simulink model "adaptive"  (R2018b)
settings: Solver=VariableStepAuto  StartTime=0.0  StopTime=40  RelTol=1e-3
values from neighbouring files (symbols this model uses):
  ADAMS_cwd = 'C:\adams_work\three_dof'    [Controls_Plant_1.m]
  ADAMS_exec = ''    [Controls_Plant_1.m]
  ADAMS_host = 'LAPTOP-5088IVHI'    [Controls_Plant_1.m]
  ADAMS_init = ''    [Controls_Plant_1.m]
  ADAMS_inputs = 'torque1!torque2!torque3'    [Controls_Plant_1.m]
  ADAMS_outputs = 'q1m!q2m!q3m!v1!v2!v3!a1!a2!a3'    [Controls_Plant_1.m]
  ADAMS_prefix = 'Controls_Plant_1'    [Controls_Plant_1.m]
  ADAMS_static = 'no'    [Controls_Plant_1.m]
  ADAMS_sysdir = 'C:\ruanjian\Adams\'    [Controls_Plant_1.m]
settings Model: Creator=73514  LastModifiedBy=73514

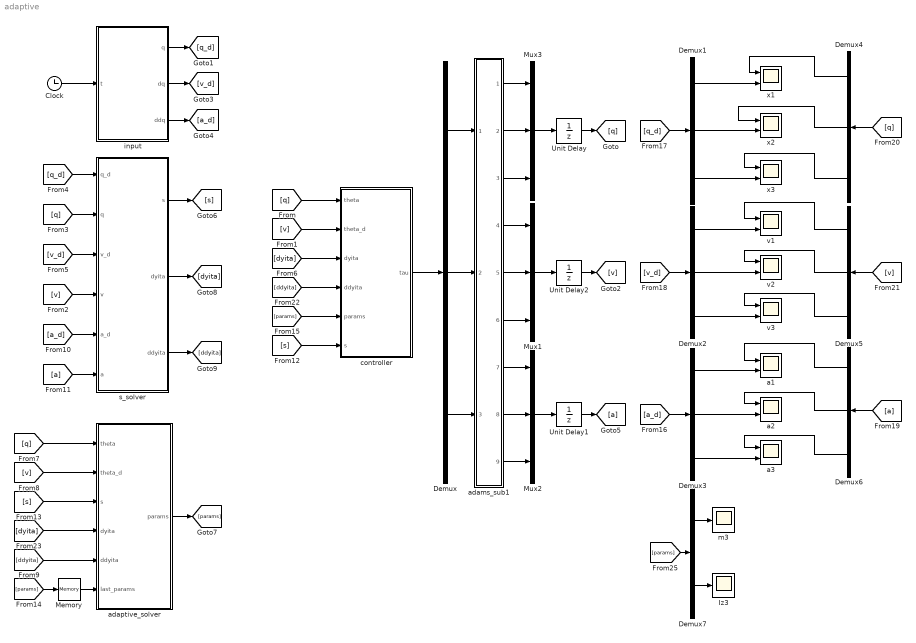
== system adaptive ==
  Clock : Clock
  Demux{,1..6} (7 alike) : Demux  Outputs=3
  Demux7 : Demux  Outputs=2
  Iz3 : Scope
  Memory : Memory  InitialCondition=[8,2]
  Mux1 : Mux  Inputs=3
  Mux2 : Mux  Inputs=3
  Mux3 : Mux  Inputs=3
  Unit Delay : UnitDelay  SampleTime=-1
  Unit Delay1 : UnitDelay  SampleTime=-1
  Unit Delay2 : UnitDelay  SampleTime=-1
  a1 : Scope  NumInputPorts=2
  a2 : Scope  NumInputPorts=2
  a3 : Scope  NumInputPorts=2
  adams_sub1 : Subsystem
  adaptive_solver : MATLAB Function  TreatAsAtomicUnit=on
  controller : MATLAB Function  TreatAsAtomicUnit=on
  input : MATLAB Function  TreatAsAtomicUnit=on
  m3 : Scope
  "s_solver " : MATLAB Function  TreatAsAtomicUnit=on
  v1 : Scope  NumInputPorts=2
  v2 : Scope  NumInputPorts=2
  v3 : Scope  NumInputPorts=2
  x1 : Scope  NumInputPorts=2
  x2 : Scope  NumInputPorts=2
  x3 : Scope  NumInputPorts=2
  wires:
  Unit Delay/1 -> [q]
  [q] -> controller/1(theta)
  Mux1/1 -> Unit Delay2/1
  Unit Delay2/1 -> [v]
  controller/1(tau) -> Demux/1
  Mux3/1 -> Unit Delay/1
  Demux/1 -> adams_sub1/1(torque1)
  [v] -> controller/2(theta_d)
  input/1(q) -> [q_d]
  input/3(ddq) -> [a_d]
  input/2(dq) -> [v_d]
  [dyita] -> controller/3(dyita)
  [q] -> adaptive_solver/1(theta)
  [v] -> adaptive_solver/2(theta_d)
  Unit Delay1/1 -> [a]
  Mux2/1 -> Unit Delay1/1
  [dyita] -> adaptive_solver/4(dyita)
  Clock/1 -> input/1(t)
  [q_d] -> "s_solver "/1(q_d)
  [q] -> "s_solver "/2(q)
  [v_d] -> "s_solver "/3(v_d)
  [v] -> "s_solver "/4(v)
  [a_d] -> "s_solver "/5(a_d)
  [a] -> "s_solver "/6(a)
  "s_solver "/1(s) -> [s]
  [s] -> controller/6(s)
  [s] -> adaptive_solver/3(s)
  adaptive_solver/1(params) -> [params]
  [params] -> controller/5(params)
  [params] -> Memory/1
  Memory/1 -> adaptive_solver/6(last_params)
  Demux/2 -> adams_sub1/2(torque2)
  Demux/3 -> adams_sub1/3(torque3)
  [v_d] -> Demux2/1
  [a_d] -> Demux3/1
  [q_d] -> Demux1/1
  adams_sub1/1(q1m) -> Mux3/1
  adams_sub1/2(q2m) -> Mux3/2
  adams_sub1/3(q3m) -> Mux3/3
  adams_sub1/4("v1 ") -> Mux1/1
  adams_sub1/5("v2 ") -> Mux1/2
  adams_sub1/6("v3 ") -> Mux1/3
  adams_sub1/7("a1 ") -> Mux2/1
  adams_sub1/8("a2 ") -> Mux2/2
  adams_sub1/9("a3 ") -> Mux2/3
  [v] -> Demux5/1
  [q] -> Demux4/1
  [a] -> Demux6/1
  Demux1/1 -> x1/2
  Demux1/2 -> x2/2
  Demux1/3 -> x3/2
  Demux2/1 -> v1/2
  Demux2/2 -> v2/2
  Demux2/3 -> v3/2
  Demux3/1 -> a1/2
  Demux3/2 -> a2/2
  Demux3/3 -> a3/2
  Demux4/1 -> x1/1
  Demux4/2 -> x2/1
  Demux4/3 -> x3/1
  Demux5/1 -> v1/1
  Demux5/2 -> v2/1
  Demux5/3 -> v3/1
  Demux6/1 -> a1/1
  Demux6/2 -> a2/1
  Demux6/3 -> a3/1
  "s_solver "/2(dyita) -> [dyita]
  "s_solver "/3(ddyita) -> [ddyita]
  [ddyita] -> controller/4(ddyita)
  [ddyita] -> adaptive_solver/5(ddyita)
  [params] -> Demux7/1
  Demux7/1 -> m3/1
  Demux7/2 -> Iz3/1

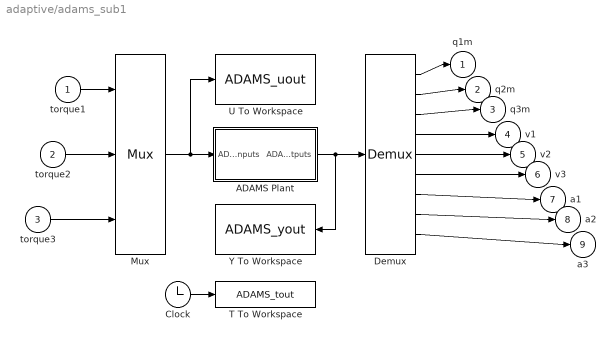
== system adaptive/adams_sub1 ==
  torque1 : Inport
  torque2 : Inport  Port=2
  torque3 : Inport  Port=3
  ADAMS Plant : Subsystem  LoadFcn=|  InitFcn=clear mex  mask(Adams Plant){exevie=ADAMS_sysdir, nam_in=ADAMS_inputs, namout=ADAMS_outputs, nampre=ADAMS_prefix, outfil=ADAMS_prefix, exesol=ADAMS_exec, stat=ADAMS_static, inicmd=[ADAMS_init], exetyp=C++, comtyp=PIPE(DDE), workdir=ADAMS_cwd, ada_host=ADAMS_host, modani=batch, modsim=discrete, dft=no, simulink_lead_cosim=yes, pin_interp_order=0, pout_extrap_order=0, pin_extrap_order=0, pout_interp_order=0, dt_out=0.005, o_rate=1, more=off}
      | %check based on dialog box setting for when setting by popup menu                                             
      | if exist('ADAMS_solver_type')                                                                                 
      |   if strcmp(ADAMS_solver_type,'C++')                                                                          
      |     set_param(gcb,'exetyp','C++');                                                                            
      |   else                                                                                                        
      |     set_param(gcb,'exetyp','Fortran');                                                                        
      |   end                                                                                                         
      | else                                                                                                          
      |   set_param(gcb,'exetyp','C++');                                                                              
      | end                                                                                                           
      | %set the mode if using acar_solver                                                                            
      | %REQUIRED HERE BECAUSE BELOW CAUSES MDLTERMINATE TO BE CALLED 2 TIMES IN MIDDLE OF SIMULATION WHEN SET IN MASK
      |                                                                                                               
      | %enable the direct feedthrough, sim mode, anim mode parameters by default                                     
      |                                                                                                               
      | if exist('set_some_params_states')                                                                            
      |                                                                                                               
      |   set_some_params_states({'dft','modsim','modani'},{'on','on','on'},'MaskEnables',gcb)                        
      |   %turn on direct feedthrough option                                                                          
      |   set_some_params_states({'dft'},{'on'},'MaskVisibilities',gcb)                                               
      |                                                                                                               
      |  end                                                                                                          
      |                                                                                                               
      |                                                                                                               
      | if exist('ADAMS_exec')                                                                                        
      |   if and(strcmp(get_param(gcb,'exesol'),'ADAMS_exec'),strcmp(ADAMS_exec,'acar_solver'))                       
      |     %set the sim mode to discrete -- only supported mode                                                      
      |     set_param(gcb,'modsim','discrete')                                                                        
      |      %turn off direct feedthrough option                                                                      
      |      set_some_params_states({'dft'},{'off'},'MaskVisibilities',gcb)                                           
      |     %set the animation mode to batch -- only supported mode                                                   
      |     set_param(gcb,'modani','batch')                                                                           
      |     %disable the direct feedthrough, sim mode, anim mode parameters                                           
      |     set_some_params_states({'modsim','modani'},{'off','off'},'MaskEnables',gcb)                               
      |   end
      |   if and(strcmp(get_param(gcb,'exesol'),'ADAMS_exec'),strcmp(ADAMS_exec,'apre_solver'))                       
      |     %set the sim mode to discrete -- only supported mode                                                      
      |     set_param(gcb,'modsim','discrete')                                                                        
      |      %turn off direct feedthrough option                                                                      
      |      set_some_params_states({'dft'},{'off'},'MaskVisibilities',gcb)                                           
      |     %set the animation mode to batch -- only supported mode                                                   
      |     set_param(gcb,'modani','batch')                                                                           
      |     %disable the direct feedthrough, sim mode, anim mode parameters                                           
      |     set_some_params_states({'modsim','modani'},{'off','off'},'MaskEnables',gcb)                               
      |   end                                                                                                  
      | end
      mask prompts: exevie "Adams install directory"; nam_in "Adams View input names"; namout "Adams View output names"; nampre "Adams model file prefix"; outfil "Output files prefix (opt.: if blank - no output)"; exesol "User executable (opt.: if blank - use standard)"; stat "Initial static simulation flag"; inicmd "Initialization commands"; exetyp "Adams Solver type"; comtyp "Interprocess option"; workdir "Adams working directory"; ada_host "Adams host"; modani "Animation mode"; modsim "Simulation mode"; dft "Direct feedthrough"; simulink_lead_cosim "Discrete Computational Order - Simulink Leads Adams"; pin_interp_order "Plant input interpolation order"; pout_extrap_order "Plant output extrapolation order"; pin_extrap_order "Plant input extrapolation order"; pout_interp_order "Plant output interpolation order"; dt_out "Communication interval"; o_rate "Number of communications per output step"; more "More parameters"
      mask help: Simulate any Adams plant model either in Adams Solver form (.adm file) or in Adams View form (.cmd file)
      settings: OpenFcn=|
      | open_system(gcb,'mask')
      | if not(exist('set_some_params_states'))
      | 
      | warning('The script "set_some_params_states.m" cannot be found in the MATLAB PATH.  Cannot update the ADAMS Plant S-Function parameters.')
      | 
      | warning('Recommended action(optional):  run the Adams Controls .m file first to help choose the correct settings in the Adams S-Function block.')
      | 
      | end
      mask Help:
      | <html>
      | This S-Function represents the non-linear Adams Plant with the inputs sent to the Adams model <br>
      |  and the outputs generated by the Adams model.  See the Adams Controls documentation for more <br>
      | information.  This plant uses the following variables:<br>
      | <br>
      | <b>ADAMS_sysdir  :</b> Adams installation directory<br>
      | <b>ADAMS_inputs  :</b> Input variables View names vector<br>
      | <b>ADAMS_outputs :</b> Outputs variables View names vector<br>
      | <b>ADAMS_prefix  : </b>ADAMS model files prefix (.adm, .cmd); also doubles as output files prefix<br>
      | <b>ADAMS_exec :</b> Adams Solver user library or keyword (e.g., acar_solver)<br>
      | <b>ADAMS_static :</b> yes|no - initial static before Co-simulation(discrete)/Function Evaluation(continuous)<br>
      | <b>ADAMS_init :</b>Initialization commands (i.e., Adams View or Solver commands, depending on setting for Animation mode)<br>
      | <b>ADAMS_cwd : </b> Current working directory (for TCP/IP)<br>
      | <b>ADAMS_host : </b>Name of Adams server host (for TCP/IP)<br>
      | <b>ADAMS_mode :</b> Linear or non-linear (i.e., co-sim, function eval)<br>
      | <b>ADAMS_solver_type :</b>Fortran or C++ (used to set popup menu when first loaded) <br>
      | 
      | 
      | <br>
      | The following settings can be chosen:<br>
      | <br>
      | <b>Adams Solver type:</b>  Fortran or C++ (will also set ADAMS_solver_type)<br>
      | <b>Interprocess option:</b> Pipe(DDE), TCP/IP or DIRECT; TCP/IP can allow different machines run Adams and MATLAB<br>
      | <b>Animation mode:</b> batch (Solver, uses .adm) or interactive (View, uses .cmd)<br>
      | <b>Simulation mode:</b> discrete (Co-simulation) or continuous (Function Evaluation)<br>
      | <b>Discrete Computational Order - Simulink Lead Adams:</b> for discrete mode, chooses if Simulink leads the integration (yes) or lags (no);<br> if set to "no", can remove algebraic loop<br>
      | <b>Plant input interpolation order:</b> 0 = zero-order hold; 1 = linear (discrete mode only, where Simulink leads)<br>
      | <b>Plant output extrapolation order:</b> 0 = zero-order hold;1 = linear(discrete mode only, where Simulink leads)<br>
      | <b>Plant input extrapolation order:</b> 0 = zero-order hold; 1 = linear (discrete mode only, where Adams leads)<br>
      | <b>Plant output interpolation order:</b> 0 = zero-order hold;1 = linear(discrete mode only, where Adams leads)<br>
      | <b>Direct feedthrough:</b> yes|no - yes = Input directly effect output(continuous mode-only)<br>
      | <b>Communication interval:</b> Time step at which Co-simulation exchange information (e.g.,0.005); also controls <br>output for continuous mode (Function Evaluation)<br>
      | <b>Number of communications per output step: </b>Sets Adams output rate (.res, .req, .gra) integer value (default: 1)<br>
      | </html>
      mask Callback exesol:
      | if exist('set_some_params_states')
      | %enable the direct feedthrough, sim mode, anim mode parameters
      | set_some_params_states({'dft','modsim','modani'},{'on','on','on'},'MaskEnables',gcb)
      | %turn on direct feedthrough option
      | set_some_params_states({'dft'},{'on'},'MaskVisibilities',gcb)
      | end
      | 
      | if exist('ADAMS_exec')
      |   if and(strcmp(get_param(gcb,'exesol'),'ADAMS_exec'),strcmp(ADAMS_exec,'acar_solver'))
      |     %set the sim mode to discrete -- only supported mode
      |     %REMOVED:  BELOW CAUSES MDLTERMINATE TO BE CALLED 2 TIMES IN MIDDLE OF SIMULATION
      |     %Now in LoadFcn callback
      |     %set_param(gcb,'modsim','discrete')
      |      %turn off direct feedthrough option
      |     set_some_params_states({'dft'},{'off'},'MaskVisibilities',gcb)
      |     %set the animation mode to batch -- only supported mode
      |     %REMOVED:  BELOW CAUSES MDLTERMINATE TO BE CALLED 2 TIMES IN MIDDLE OF SIMULATION
      |     %Now in LoadFcn callback
      |     %set_param(gcb,'modani','batch')
      |     %disable the direct feedthrough, sim mode, anim mode parameters
      |     set_some_params_states({'modsim','modani'},{'off','off'},'MaskEnables',gcb)
      |   end
      | end
      mask TypeOptions exetyp: Fortran | C++
      mask Callback exetyp:
      | if strcmp(get_param(gcb,'exetyp'),'C++')
      |     ADAMS_solver_type='C++';
      | else
      |     ADAMS_solver_type='Fortran';
      | end
      mask TypeOptions comtyp: PIPE(DDE) | TCP/IP | DIRECT
      mask Callback comtyp:
      | if exist('set_some_params_states')
      | if strcmp(get_param(gcb,'comtyp'),'PIPE(DDE)') || strcmp(get_param(gcb,'comtyp'),'DIRECT')
      |     %turn off cwd, host options
      |     set_some_params_states({'ada_host','workdir'},{'off','off'},'MaskVisibilities',gcb)
      | else%if strcmp(get_param(gcb,'modsim'),'TCP/IP')
      |     %turn on cwd, host options
      |     set_some_params_states({'ada_host','workdir'},{'on','on'},'MaskVisibilities',gcb)
      | end
      | end
      mask TypeOptions modani: batch | interactive
      mask TypeOptions modsim: discrete | continuous
      mask Callback modsim:
      | if exist('set_some_params_states')
      | if strcmp(get_param(gcb,'modsim'),'discrete')
      |      %turn off direct feedthrough option
      |     set_some_params_states({'dft'},{'off'},'MaskVisibilities',gcb)
      |     %turn on discrete co-sim type if want to see more
      |     if strcmp(get_param(gcb,'more'),'on')
      |         set_some_params_states({'simulink_lead_cosim'},{'on'},'MaskVisibilities',gcb)
      |     end
      |     if strcmp(get_param(gcb,'simulink_lead_cosim'),'yes')
      |         %turn on interpolation/extrapolation options
      |         set_some_params_states({'pin_interp_order','pout_extrap_order',},{'on','on'},'MaskVisibilities',gcb)
      |     else
      |         set_some_params_states({'pin_extrap_order','pout_interp_order'},{'on','on'},'MaskVisibilities',gcb)
      |     end
      | else%if strcmp(get_param(gcb,'modsim'),'continuous')
      |      %turn off direct feedthrough option
      |     set_some_params_states({'dft'},{'on'},'MaskVisibilities',gcb)
      |     %turn off interpolation/extrapolation options
      |     set_some_params_states({'pin_interp_order','pout_extrap_order','pin_extrap_order','pout_interp_order','simulink_lead_cosim'},{'off','off','off','off','off'},'MaskVisibilities',gcb)
      | end
      | end
      mask TypeOptions dft: no | yes
      mask TypeOptions simulink_lead_cosim: yes | no
      mask Callback simulink_lead_cosim:
      | if exist('set_some_params_states')
      | if (strcmp(get_param(gcb,'simulink_lead_cosim'),'yes') && strcmp(get_param(gcb,'modsim'),'discrete'))
      |      %turn off unused interpolate/extrapolate options
      |     set_some_params_states({'pin_extrap_order','pout_interp_order'},{'off','off'},'MaskVisibilities',gcb)
      |     %turn on used interpolate/extrapolate options
      |     set_some_params_states({'pin_interp_order','pout_extrap_order'},{'on','on'},'MaskVisibilities',gcb)
      | elseif (strcmp(get_param(gcb,'simulink_lead_cosim'),'no') && strcmp(get_param(gcb,'modsim'),'discrete'))
      |     %turn on used interpolate/extrapolate options
      |     set_some_params_states({'pin_extrap_order','pout_interp_order'},{'on','on'},'MaskVisibilities',gcb)
      |      %turn off unused interpolate/extrapolate options
      |     set_some_params_states({'pin_interp_order','pout_extrap_order'},{'off','off'},'MaskVisibilities',gcb)
      | end
      | end
      mask TypeOptions pin_interp_order: 0 | 1
      mask TypeOptions pout_extrap_order: 0 | 1
      mask TypeOptions pin_extrap_order: 0 | 1
      mask TypeOptions pout_interp_order: 0 | 1
      mask Callback more:
      | if exist('set_some_params_states')
      | if (strcmp(get_param(gcb,'more'),'on'))
      |      %turn on infrequently used options
      |     set_some_params_states({'exevie','nam_in','namout','exesol','stat','inicmd'},{'on','on','on','on','on','on'},'MaskVisibilities',gcb)
      |     if strcmp(get_param(gcb,'modsim'),'discrete')
      |         set_some_params_states({'simulink_lead_cosim'},{'on'},'MaskVisibilities',gcb)
      |     end
      | elseif (strcmp(get_param(gcb,'more'),'off'))
      |     %turn off infrequently used options
      |     set_some_params_states({'exevie','nam_in','namout','exesol','stat','inicmd'},{'off','off','off','off','off','off'},'MaskVisibilities',gcb)
      |     if strcmp(get_param(gcb,'modsim'),'discrete')
      |         set_some_params_states({'simulink_lead_cosim'},{'off'},'MaskVisibilities',gcb)
      |     end
      | end
      | end
      mask Display: disp( 'MSC Software' )
  Clock : Clock
  Demux : Demux  Outputs=9
  Mux : Mux  Inputs=3
  T To Workspace : ToWorkspace  VariableName=ADAMS_tout
      settings: MaxDataPoints=100000
  U To Workspace : ToWorkspace  VariableName=ADAMS_uout
      settings: MaxDataPoints=100000
  Y To Workspace : ToWorkspace  VariableName=ADAMS_yout
      settings: MaxDataPoints=100000
  q1m : Outport
  q2m : Outport  Port=2
  q3m : Outport  Port=3
  "v1 " : Outport  Port=4
  "v2 " : Outport  Port=5
  "v3 " : Outport  Port=6
  "a1 " : Outport  Port=7
  "a2 " : Outport  Port=8
  "a3 " : Outport  Port=9
  wires:
  Clock/1 -> T To Workspace/1
  Mux/1 -> ADAMS Plant/1(ADAMS inputs), U To Workspace/1
  ADAMS Plant/1(ADAMS outputs) -> Demux/1, Y To Workspace/1
  Demux/1 -> q1m/1
  Demux/2 -> q2m/1
  Demux/3 -> q3m/1
  Demux/4 -> "v1 "/1
  Demux/5 -> "v2 "/1
  Demux/6 -> "v3 "/1
  Demux/7 -> "a1 "/1
  Demux/8 -> "a2 "/1
  Demux/9 -> "a3 "/1
  torque1/1 -> Mux/1
  torque2/1 -> Mux/2
  torque3/1 -> Mux/3

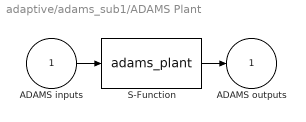
== system adaptive/adams_sub1/ADAMS Plant ==
  ADAMS inputs : Inport
  S-Function : S-Function  StopFcn=clear mex  FunctionName=adams_plant  Parameters=exevie,exesol,stat,outfil,nampre,o_rate,nam_in,namout,dft,modsim,modani,dt_out,inicmd,exetyp,comtyp,ada_host, workdir,pin_interp_order,pout_extrap_order,pin_extrap_order,pout_interp_order,simulink_lead_cosim  SFunctionDeploymentMode=off  EnableBusSupport=off
  ADAMS outputs : Outport  InitialOutput=0
  wires:
  ADAMS inputs/1 -> S-Function/1
  S-Function/1 -> ADAMS outputs/1

== matlab function adaptive/adaptive_solver ==
  data: theta input; params output; theta_d input; s input; dyita input; ddyita input; last_params input
function params = adaptive_solver(theta, theta_d,s,dyita,ddyita,last_params)
dq1=theta_d(1);dq2=theta_d(2);dq3=theta_d(3);
q1=theta(1);q2=theta(2);q3=theta(3);
dyita1=dyita(1);dyita2=dyita(2);dyita3=dyita(3);
ddyita1=ddyita(1);ddyita2=ddyita(2);ddyita3=ddyita(3);
%杆长和质心位置
d1=1; d2=1; d3=1;
xc1=0.5;xc2=0.5;xc3=0.5;
%质量与惯量矩阵
m3=last_params(1);
Iz3=last_params(2);
w=zeros(3,2);
w(1,2)=ddyita1+ddyita2+ddyita3;
w(2,2)=ddyita1+ddyita2+ddyita3;
w(3,2)=ddyita1+ddyita2+ddyita3;
w(1,1)=ddyita3*(d2*xc3*cos(q3) + d1*xc3*cos(q2 + q3)) - dyita2*(d1*dq1*(xc3*sin(q2 + q3) + d2*sin(q2)) + d1*dq2*(xc3*sin(q2 + q3) + d2*sin(q2)) + dq3*xc3*(d1*sin(q2 + q3) + d2*sin(q3))) - dyita1*(dq2*(d1*d2*sin(q2) + d1*xc3*sin(q2 + q3)) + dq3*(d2*xc3*sin(q3) + d1*xc3*sin(q2 + q3))) + ddyita1*(d1^2 + 2*cos(q2)*d1*d2 + 2*xc3*cos(q2 + q3)*d1 + d2^2 + 2*xc3*cos(q3)*d2) + ddyita2*(d2^2 + 2*d2*xc3*cos(q3) + d1*xc3*cos(q2 + q3) + d1*d2*cos(q2)) - dyita3*xc3*(d1*sin(q2 + q3) + d2*sin(q3))*(dq1 + dq2 + dq3);
w(2,1)=dyita1*(dq1*(d1*d2*sin(q2) + d1*xc3*sin(q2 + q3)) - d2*dq3*xc3*sin(q3)) + ddyita1*(d2^2 + 2*d2*xc3*cos(q3) + d1*xc3*cos(q2 + q3) + d1*d2*cos(q2)) + ddyita2*(d2^2 + 2*xc3*cos(q3)*d2) + d2*ddyita3*xc3*cos(q3) - d2*dyita3*xc3*sin(q3)*(dq1 + dq2 + dq3) - d2*dq3*dyita2*xc3*sin(q3);
w(3,1)=ddyita1*(d2*xc3*cos(q3) + d1*xc3*cos(q2 + q3)) + dyita1*(dq1*(d2*xc3*sin(q3) + d1*xc3*sin(q2 + q3)) + d2*dq2*xc3*sin(q3)) + d2*ddyita2*xc3*cos(q3) + d2*dyita2*xc3*sin(q3)*(dq1 + dq2);
%自适应率
gamma=1;
phi=-gamma*w'*s;
m3=m3-phi(1);
Iz3=Iz3-phi(2);
params=[m3,Iz3];
end

== matlab function adaptive/controller ==
  data: theta input; tau output; theta_d input; dyita input; ddyita input; params input; s input
function tau = controller(theta, theta_d, dyita,ddyita, params, s)
tau=zeros(3,1);
dq1=theta_d(1);dq2=theta_d(2);dq3=theta_d(3);
q1=theta(1);q2=theta(2);q3=theta(3);
%杆长和质心位置
d1=1; d2=1; d3=1;
xc1=0.5;xc2=0.5;xc3=0.5;
%质量与惯量矩阵
m1=10;m2=10;m3=params(1);
Iz1=1.05+m1*xc1^2;Iz2=1.05+m2*xc2^2;Iz3=params(2);
%计算
k=100;

h=[ Iz1 + Iz2 + Iz3 + d1^2*m2 + d1^2*m3 + d2^2*m3 + 2*d1*m3*xc3*cos(q2 + q3) + 2*d1*d2*m3*cos(q2) + 2*d1*m2*xc2*cos(q2) + 2*d2*m3*xc3*cos(q3), Iz2 + Iz3 + d2^2*m3 + d1*m3*xc3*cos(q2 + q3) + d1*d2*m3*cos(q2) + d1*m2*xc2*cos(q2) + 2*d2*m3*xc3*cos(q3), Iz3 + d1*m3*xc3*cos(q2 + q3) + d2*m3*xc3*cos(q3);
                                 Iz2 + Iz3 + d2^2*m3 + d1*m3*xc3*cos(q2 + q3) + d1*d2*m3*cos(q2) + d1*m2*xc2*cos(q2) + 2*d2*m3*xc3*cos(q3),                                                                 m3*d2^2 + 2*m3*xc3*cos(q3)*d2 + Iz2 + Iz3,                          Iz3 + d2*m3*xc3*cos(q3);
                                                                                          Iz3 + d1*m3*xc3*cos(q2 + q3) + d2*m3*xc3*cos(q3),                                                                                   Iz3 + d2*m3*xc3*cos(q3),                                              Iz3];

c=[ - dq3*(d1*m3*xc3*sin(q2 + q3) + d2*m3*xc3*sin(q3)) - dq2*(d1*m3*xc3*sin(q2 + q3) + d1*d2*m3*sin(q2) + d1*m2*xc2*sin(q2)), - d1*dq1*(d2*m3*sin(q2) + m2*xc2*sin(q2) + m3*xc3*sin(q2 + q3)) - d1*dq2*(d2*m3*sin(q2) + m2*xc2*sin(q2) + m3*xc3*sin(q2 + q3)) - dq3*m3*xc3*(d1*sin(q2 + q3) + d2*sin(q3)), -m3*xc3*(d1*sin(q2 + q3) + d2*sin(q3))*(dq1 + dq2 + dq3);
                              dq1*(d1*m3*xc3*sin(q2 + q3) + d1*d2*m3*sin(q2) + d1*m2*xc2*sin(q2)) - d2*dq3*m3*xc3*sin(q3),                                                                                                                                                      -d2*dq3*m3*xc3*sin(q3),                     -d2*m3*xc3*sin(q3)*(dq1 + dq2 + dq3);
                                                 dq1*(d1*m3*xc3*sin(q2 + q3) + d2*m3*xc3*sin(q3)) + d2*dq2*m3*xc3*sin(q3),                                                                                                                                               d2*m3*xc3*sin(q3)*(dq1 + dq2),                                                        0];
tau=h*ddyita+c*dyita+k*s;
end

== matlab function adaptive/input ==
  data: t input; q output; dq output; ddq output
function [q,dq,ddq] = input(t)
q=zeros(3,1);
dq=zeros(3,1);
ddq=zeros(3,1);
%等加速度输入信号
%k=0.01;
%a=2*k;
%v=2*k*t;
%x=k*t^2;
%正弦输入信号
k=0.01;w=3;
x=k*(1-cos(w*t));
v=w*k*sin(w*t);
a=w^2*k*cos(w*t);
q=[x;x;x];
dq=[v;v;v];
ddq=[a;a;a];

end

== matlab function adaptive/s_solver  ==
  data: q_d input; s output; dyita output; ddyita output; q input; v_d input; v input; a_d input; a input
function [s,dyita,ddyita] = s_solver(q_d,q,v_d,v,a_d,a)
lamuda=4;
e=q_d-q;
de=v_d-v;
s=de+lamuda*e;
dyita=v_d+lamuda*e;
ddyita=a_d+lamuda*de;

end
